simulink model "Gain_TestGen18"  (R2017b)
settings: Solver=FixedStepDiscrete  StartTime=0.0  StopTime=10.0  RelTol=1e-3
undefined symbols (not defined in the file): Block_TestLib, enable
settings Model: Creator=ktrinh  LastModifiedBy=ktrinh
settings DebuggingCC: ParameterOverflowMsg=none

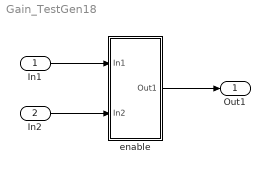
== system Gain_TestGen18 ==
  In1 : Inport
  In2 : Inport  Port=2
  enable : Subsystem  AncestorBlock=Block_TestLib/enable
  Out1 : Outport
  wires:
  In1/1 -> enable/1(In1)
  In2/1 -> enable/2(In2)
  enable/1(Out1) -> Out1/1

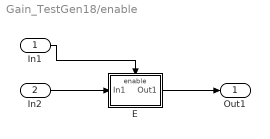
== system Gain_TestGen18/enable ==
  In1 : Inport  OutDataTypeStr=boolean
  In2 : Inport  Port=2
  E : Subsystem  TreatAsAtomicUnit=on
  Out1 : Outport
  wires:
  In1/1 -> E/Enable
  In2/1 -> E/1(In1)
  E/1(Out1) -> Out1/1

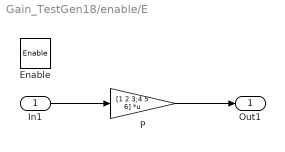
== system Gain_TestGen18/enable/E ==
  In1 : Inport  PortDimensions=[3,2]
  Enable : EnablePort
  P : Gain  Gain=[1 2 3;4 5 6]  Multiplication=Matrix(K*u)  ParamDataTypeStr=uint16  OutMin=1.  OutMax=100  OutDataTypeStr=int16  RndMeth=Nearest  SaturateOnIntegerOverflow=on  LockScale=on
  Out1 : Outport
  wires:
  In1/1 -> P/1
  P/1 -> Out1/1
